simulink model "sim_IDCS"  (R2020a)
settings: Solver=ode4  StartTime=0  StopTime=t_end  FixedStep=Step_Time  RelTol=1e-3
values from neighbouring files (symbols this model uses):
  A = [ 0 0 1 0 ... (first row only)    [bode_IDCS.m]    (also in bode_hiratsuka_IDCS.m = 1; hiratsuka_IDCS.m = 0.003; model_IDCS.m = 0.003; model_hiratsuka_nondamper.m = 0.003)
  c1 = 150    [bode_hiratsuka_IDCS.m]    (also in hiratsuka_IDCS.m = 5; model_IDCS.m = 5; model_hiratsuka_nondamper.m = 15; model_linear_damper.m = 50)
  c2 = 7    [bode_IDCS.m]    (also in bode_hiratsuka_IDCS.m; hiratsuka_IDCS.m; model_IDCS.m; model_hiratsuka_nondamper.m)
  Hz = wv(k)    [bode_hiratsuka_IDCS.m]    (also in hiratsuka_IDCS.m = 6.28318530718; model_IDCS.m = 6.28318530718; model_hiratsuka_nondamper.m = 6.28318530718; model_linear_damper.m = 31.4159265359)
  k1 = 2200    [bode_IDCS.m]    (also in bode_hiratsuka_IDCS.m; hiratsuka_IDCS.m; model_IDCS.m; model_hiratsuka_nondamper.m)
  k2 = 405    [bode_IDCS.m]    (also in bode_hiratsuka_IDCS.m; hiratsuka_IDCS.m; model_IDCS.m; model_hiratsuka_nondamper.m)
  Kp = 10    [bode_IDCS.m]    (also in bode_hiratsuka_IDCS.m = 80; hiratsuka_IDCS.m = 60; model_IDCS.m = 100; model_hiratsuka_nondamper.m = 80)
  m1 = 1.5    [bode_IDCS.m]    (also in bode_hiratsuka_IDCS.m; hiratsuka_IDCS.m; model_IDCS.m; model_hiratsuka_nondamper.m)
  m2 = 6.4    [bode_IDCS.m]    (also in bode_hiratsuka_IDCS.m; hiratsuka_IDCS.m; model_IDCS.m; model_hiratsuka_nondamper.m)
  T_diff = 1/(2*pi*cutoff)    (= 0.00795774715459)    [bode_IDCS.m]    (also in hiratsuka_IDCS.m = 0.00159154943092; model_IDCS.m = 0.00159154943092; model_hiratsuka_nondamper.m = 0.00159154943092; model_linear_damper.m)
undefined symbols (not defined in the file or in its folder): Kd, Ki
libraries: simulink x1
settings Model: Creator=Peanatsu  LastModifiedBy=Natsu Nakagawa

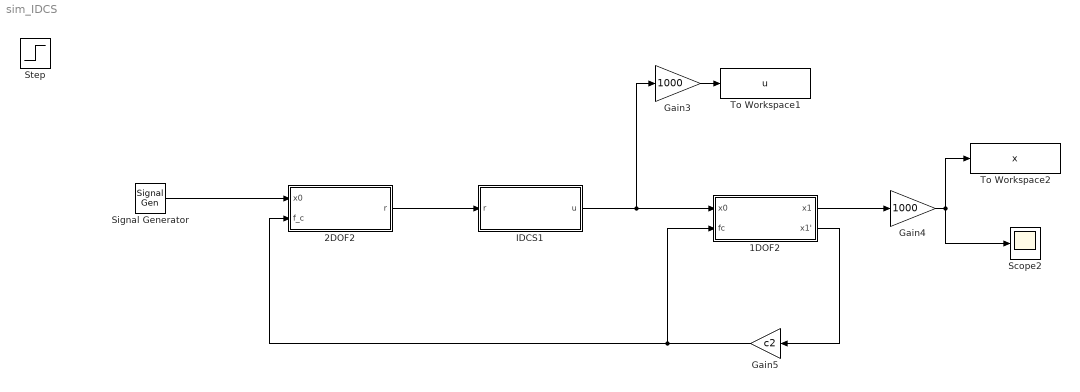
== system sim_IDCS ==
  1DOF2 : Subsystem
  2DOF2 : Subsystem
  Gain3 : Gain  Gain=1000
  Gain4 : Gain  Gain=1000
  Gain5 : Gain  Gain=c2
  IDCS1 : Subsystem
  Scope2 : Scope
  Signal Generator : SignalGenerator  Amplitude=A  Frequency=Hz  Units=rad/sec
  Step : Step  After=A  SampleTime=0
  To Workspace1 : ToWorkspace  VariableName=u  SaveFormat=Timeseries  SampleTime=-1
  To Workspace2 : ToWorkspace  VariableName=x  SaveFormat=Timeseries  SampleTime=-1
  wires:
  IDCS1/1(u) -> Gain3/1, 1DOF2/1(x0)
  Gain4/1 -> To Workspace2/1, Scope2/1
  2DOF2/1(r) -> IDCS1/1(r)
  1DOF2/1(x1) -> Gain4/1
  1DOF2/2(x1') -> Gain5/1
  Gain3/1 -> To Workspace1/1
  Signal Generator/1 -> 2DOF2/1(x0)
  Gain5/1 -> 2DOF2/2(f_c), 1DOF2/2(fc)

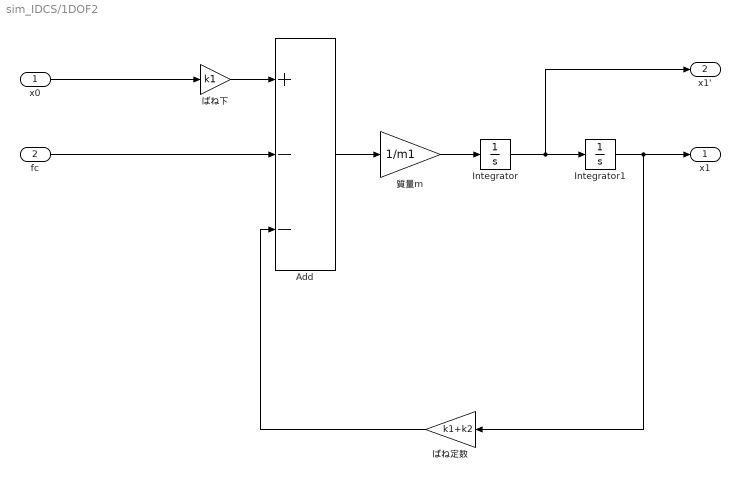
== system sim_IDCS/1DOF2 ==
  x0 : Inport
  fc : Inport  Port=2
  Add : Sum  Inputs=+--
  Integrator : Integrator
  Integrator1 : Integrator
  ばね下 : Gain  Gain=k1
  "ばね定数 " : Gain  Gain=k1+k2
  質量m : Gain  Gain=1/m1
  x1 : Outport
  x1' : Outport  Port=2
  wires:
  Integrator/1 -> Integrator1/1, x1'/1
  Add/1 -> 質量m/1
  x0/1 -> ばね下/1
  質量m/1 -> Integrator/1
  Integrator1/1 -> x1/1, "ばね定数 "/1
  ばね下/1 -> Add/1
  "ばね定数 "/1 -> Add/3
  fc/1 -> Add/2

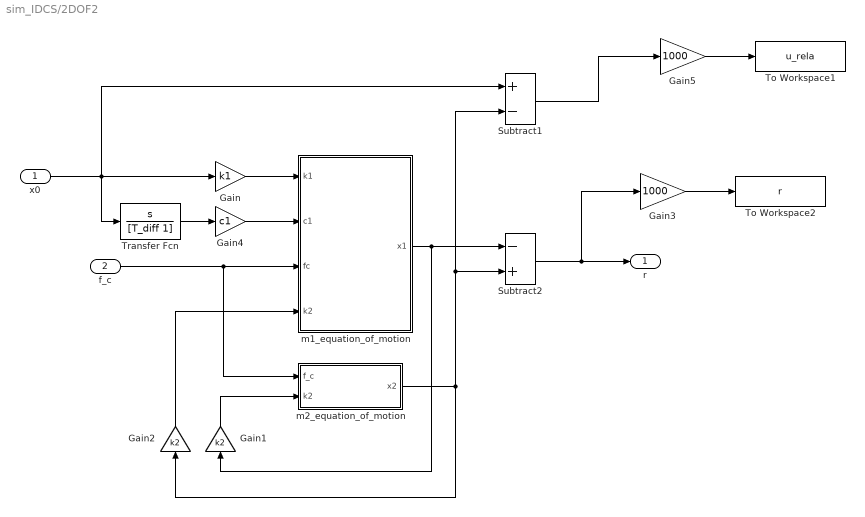
== system sim_IDCS/2DOF2 ==
  x0 : Inport
  f_c : Inport  Port=2
  Gain : Gain  Gain=k1
  Gain1 : Gain  Gain=k2
  Gain2 : Gain  Gain=k2
  Gain3 : Gain  Gain=1000
  Gain4 : Gain  Gain=c1
  Gain5 : Gain  Gain=1000
  Subtract1 : Sum  Inputs=+-
  Subtract2 : Sum  Inputs=-+
  To Workspace1 : ToWorkspace  VariableName=u_rela  SaveFormat=Timeseries  SampleTime=-1
  To Workspace2 : ToWorkspace  VariableName=r  SaveFormat=Timeseries  SampleTime=-1
  Transfer Fcn : TransferFcn  Numerator=[1 0]  Denominator=[T_diff 1]
  m1_equation_of_motion : Subsystem
  m2_equation_of_motion : Subsystem
  r : Outport
  wires:
  x0/1 -> Subtract1/1, Gain/1, Transfer Fcn/1
  Gain/1 -> m1_equation_of_motion/1(k1)
  m1_equation_of_motion/1(x1) -> Gain1/1, Subtract2/1
  f_c/1 -> m2_equation_of_motion/1(f_c), m1_equation_of_motion/3(fc)
  Gain1/1 -> m2_equation_of_motion/2("k2 ")
  m2_equation_of_motion/1(x2) -> Gain2/1, Subtract1/2, Subtract2/2
  Subtract2/1 -> Gain3/1, r/1
  Gain4/1 -> m1_equation_of_motion/2(c1)
  Gain2/1 -> m1_equation_of_motion/4(k2)
  Transfer Fcn/1 -> Gain4/1
  Gain3/1 -> To Workspace2/1
  Subtract1/1 -> Gain5/1
  Gain5/1 -> To Workspace1/1

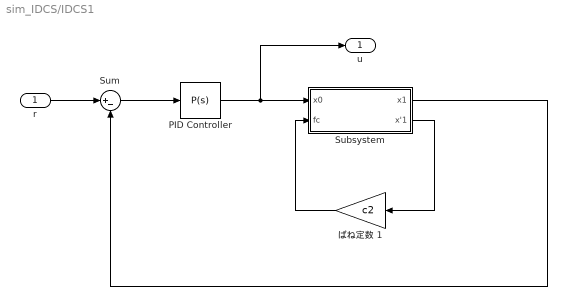
== system sim_IDCS/IDCS1 ==
  r : Inport
  PID Controller : simulink/Continuous/PID Controller  Controller=P  Form=Ideal  TimeDomain=Continuous-time  UseExternalTs=off  SampleTime=-1  IntegratorMethod=Forward Euler  FilterMethod=Forward Euler  ControllerParametersSource=internal  P=Kp  I=Ki  D=Kd  UseFilter=on  N=100  TunerSelectOption=Transfer Function Based (PID Tuner App)  InitialConditionSource=internal  InitialConditionForIntegrator=0  InitialConditionForFilter=0  DifferentiatorICPrevScaledInput=0  ExternalReset=none  TrackingMode=off  Kt=1  LimitOutput=off  UpperSaturationLimit=inf  LowerSaturationLimit=-inf  LinearizeAsGain=on  AntiWindupMode=none  Kb=1  POutMin=[]  POutMax=[]  IOutMin=[]  IOutMax=[]  DOutMin=[]  DOutMax=[]  NOutMin=[]  NOutMax=[]  SumOutMin=[]  SumOutMax=[]  SaturationOutMin=[]  SaturationOutMax=[]  PParamMin=[]  PParamMax=[]  IParamMin=[]  IParamMax=[]  DParamMin=[]  DParamMax=[]  NParamMin=[]  NParamMax=[]  KbParamMin=[]  KbParamMax=[]  KtParamMin=[]  KtParamMax=[]  KbOutMin=[]  KbOutMax=[]  KtOutMin=[]  KtOutMax=[]  IntegratorOutMin=[]  IntegratorOutMax=[]  FilterOutMin=[]  FilterOutMax=[]  SumI1OutMin=[]  SumI1OutMax=[]  SumI2OutMin=[]  SumI2OutMax=[]  SumI3OutMin=[]  SumI3OutMax=[]  SumI4OutMin=[]  SumI4OutMax=[]  SumDOutMin=[]  SumDOutMax=[]  DifferentiatorOutMin=[]  DifferentiatorOutMax=[]  FilterDiffOutCoefMin=[]  FilterDiffOutCoefMax=[]  ReciprocalOutMin=[]  ReciprocalOutMax=[]  SumDenOutMin=[]  SumDenOutMax=[]  SumNumOutMin=[]  SumNumOutMax=[]  DivideOutMin=[]  DivideOutMax=[]  UdiffTsProdOutMin=[]  UdiffTsProdOutMax=[]  NTsProdOutMin=[]  NTsProdOutMax=[]  UintegralTsProdOutMin=[]  UintegralTsProdOutMax=[]  UngainTsProdOutMin=[]  UngainTsProdOutMax=[]  IntegratorContinuousStateAttributes=''  IntegratorStateMustResolveToSignalObject=off  IntegratorRTWStateStorageClass=Auto  FilterContinuousStateAttributes=''  FilterStateMustResolveToSignalObject=off  FilterRTWStateStorageClass=Auto  ParallelPVariant=InternalParameters  IdealPVariant=Disabled  IVariant=Disabled  DVariant=Disabled  IntegratorVariant=Disabled  SatVariant=Disabled  AWVariant=Disabled  PCopyVariant=Disabled  TRVariant=Disabled  FdbkBlocksVariant=Forward  IdealPFdbkVariant=Disabled  SatFdbkVariant=Disabled  DerivativeFilterVariant=Disabled  NVariant=Disabled  NCopyVariant=Disabled_SignalSpec  FilterICVariant=Disabled  IntegratorICVariant=Disabled  ExternalResetVariant=Disabled  TRSumVariant=Passthrough  SumFdbkVariant=Disabled  SumVariant=Passthrough_P  TsampFilterVariant=InternalTs  TsampNgainVariant=Passthrough  TsampIntegralVariant=Disabled_SignalSpec
  Subsystem : Subsystem
  Sum : Sum  Inputs=|+-
  ばね定数 1 : Gain  Gain=c2
  u : Outport
  wires:
  r/1 -> Sum/1
  Sum/1 -> PID Controller/1
  PID Controller/1 -> u/1, Subsystem/1(x0)
  Subsystem/1(x1) -> Sum/2
  Subsystem/2(x'1) -> ばね定数 1/1
  ばね定数 1/1 -> Subsystem/2(fc)

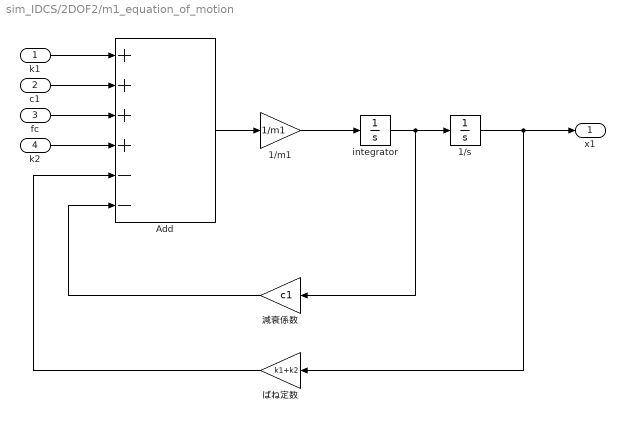
== system sim_IDCS/2DOF2/m1_equation_of_motion ==
  k1 : Inport
  c1 : Inport  Port=2
  fc : Inport  Port=3
  k2 : Inport  Port=4
  1/m1 : Gain  Gain=1/m1
  1/s : Integrator
  Add : Sum  Inputs=++++--
  integrator : Integrator
  ばね定数 : Gain  Gain=k1+k2
  減衰係数 : Gain  Gain=c1
  x1 : Outport
  wires:
  k1/1 -> Add/1
  c1/1 -> Add/2
  Add/1 -> 1/m1/1
  integrator/1 -> 1/s/1, 減衰係数/1
  1/s/1 -> x1/1, ばね定数/1
  fc/1 -> Add/3
  1/m1/1 -> integrator/1
  k2/1 -> Add/4
  ばね定数/1 -> Add/5
  減衰係数/1 -> Add/6

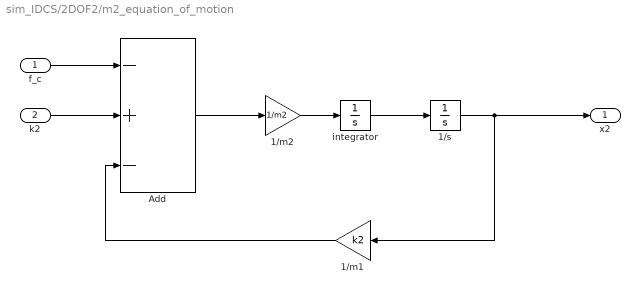
== system sim_IDCS/2DOF2/m2_equation_of_motion ==
  f_c : Inport
  "k2 " : Inport  Port=2
  1/m1 : Gain  Gain=k2
  1/m2 : Gain  Gain=1/m2
  1/s : Integrator
  Add : Sum  Inputs=-+-
  integrator : Integrator
  x2 : Outport
  wires:
  f_c/1 -> Add/1
  "k2 "/1 -> Add/2
  Add/1 -> 1/m2/1
  integrator/1 -> 1/s/1
  1/s/1 -> 1/m1/1, x2/1
  1/m1/1 -> Add/3
  1/m2/1 -> integrator/1

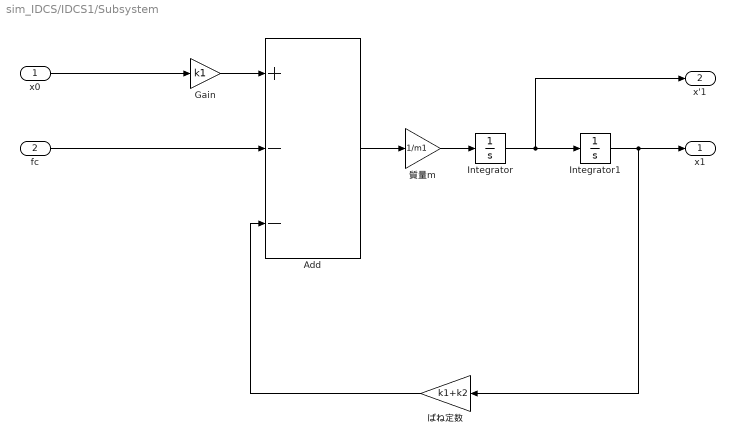
== system sim_IDCS/IDCS1/Subsystem ==
  x0 : Inport
  fc : Inport  Port=2
  Add : Sum  Inputs=+--
  Gain : Gain  Gain=k1
  Integrator : Integrator
  Integrator1 : Integrator
  "ばね定数 " : Gain  Gain=k1+k2
  質量m : Gain  Gain=1/m1
  x1 : Outport
  x'1 : Outport  Port=2
  wires:
  Integrator/1 -> x'1/1, Integrator1/1
  Add/1 -> 質量m/1
  x0/1 -> Gain/1
  質量m/1 -> Integrator/1
  Integrator1/1 -> x1/1, "ばね定数 "/1
  Gain/1 -> Add/1
  fc/1 -> Add/2
  "ばね定数 "/1 -> Add/3
